simulink model "zbr"  (Simulink 8.1)
settings: Solver=ode4  StartTime=0.0  StopTime=600  FixedStep=0.01  RelTol=1e-3
values from neighbouring files (symbols this model uses):
  T_0 = 293    [matlab.mat]
  V_0 = 0.04    [matlab.mat]
settings Model: Creator=student  LastModifiedBy=adasdeb
settings DebuggingCC: FcnCallInpInsideContextMsg=EnableAllAsWarning
settings GRTTargetCC: CombineOutputUpdateFcns=on  GRTInterface=off

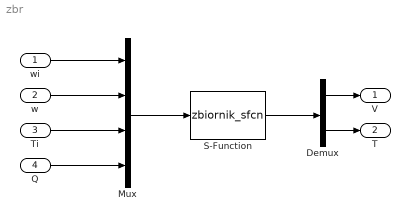
== system zbr ==
  wi : Inport
  w : Inport  Port=2
  Ti : Inport  Port=3
  Q : Inport  Port=4
  Demux : Demux  Outputs=2
  Mux : Mux
  S-Function : S-Function  FunctionName=zbiornik_sfcn  Parameters=V_0 T_0  EnableBusSupport=off
  V : Outport
  T : Outport  Port=2
  wires:
  Mux/1 -> S-Function/1
  Demux/2 -> T/1
  Demux/1 -> V/1
  Q/1 -> Mux/4
  Ti/1 -> Mux/3
  w/1 -> Mux/2
  wi/1 -> Mux/1
  S-Function/1 -> Demux/1
